simulink model "Controle_P"  (R2014a)
settings: Solver=ode45  StartTime=0.0  StopTime=1.5  RelTol=1e-3
values from neighbouring files (symbols this model uses):
  K = place(a,b,P)    [Controle_Posicao.m]
settings Model: Creator=unieerisantos  LastModifiedBy=unieerisantos
settings DataIOCC: Refine=10

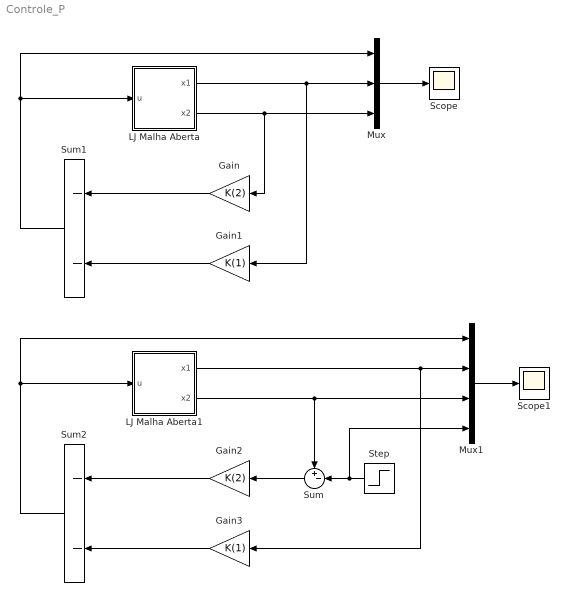
== system Controle_P ==
  Gain : Gain  Gain=K(2)
  Gain1 : Gain  Gain=K(1)
  Gain2 : Gain  Gain=K(2)
  Gain3 : Gain  Gain=K(1)
  LJ Malha Aberta : Subsystem
  LJ Malha Aberta1 : Subsystem
  Mux : Mux  Inputs=3
  Mux1 : Mux
  Scope : Scope
      settings: SaveName=ControleVcomInt
  Scope1 : Scope
  Step : Step  Time=0  After=10  SampleTime=0
  Sum : Sum  Inputs=+-|
  Sum1 : Sum  Inputs=--
  Sum2 : Sum  Inputs=--
  wires:
  LJ Malha Aberta/2("x2 ") -> Gain/1, Mux/3
  LJ Malha Aberta/1(x1) -> Gain1/1, Mux/2
  Gain/1 -> Sum1/1
  Gain1/1 -> Sum1/2
  Sum1/1 -> Mux/1, LJ Malha Aberta/1(u)
  Mux/1 -> Scope/1
  LJ Malha Aberta1/1(x1) -> Gain3/1, Mux1/2
  Gain2/1 -> Sum2/1
  Gain3/1 -> Sum2/2
  Sum2/1 -> Mux1/1, LJ Malha Aberta1/1(u)
  Mux1/1 -> Scope1/1
  LJ Malha Aberta1/2("x2 ") -> Mux1/3, Sum/1
  Sum/1 -> Gain2/1
  Step/1 -> Mux1/4, Sum/2

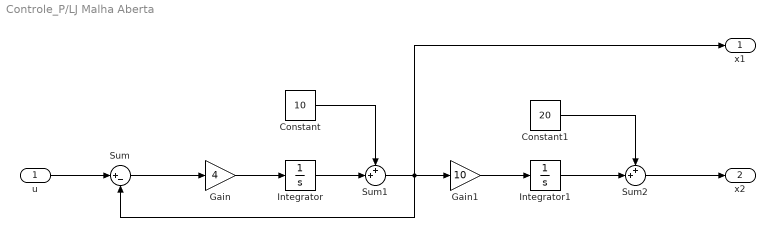
== system Controle_P/LJ Malha Aberta ==
  u : Inport
  Constant : Constant  Value=10
  Constant1 : Constant  Value=20
  Gain : Gain  Gain=4
  Gain1 : Gain  Gain=10
  Integrator : Integrator
  Integrator1 : Integrator
  Sum : Sum  Inputs=|+-
  Sum1 : Sum  Inputs=++|
  Sum2 : Sum  Inputs=++|
  x1 : Outport
  "x2 " : Outport  Port=2
  wires:
  Sum/1 -> Gain/1
  u/1 -> Sum/1
  Gain1/1 -> Integrator1/1
  Gain/1 -> Integrator/1
  Integrator/1 -> Sum1/2
  Sum1/1 -> Sum/2, x1/1, Gain1/1
  Constant/1 -> Sum1/1
  Integrator1/1 -> Sum2/2
  Constant1/1 -> Sum2/1
  Sum2/1 -> "x2 "/1

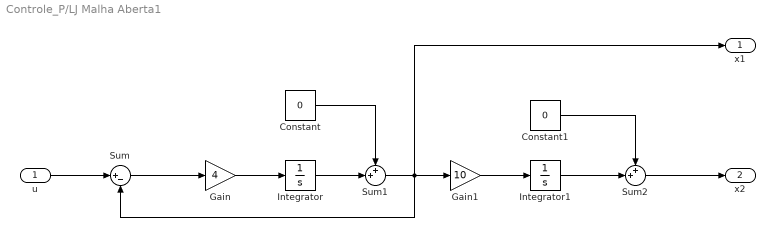
== system Controle_P/LJ Malha Aberta1 ==
  u : Inport
  Constant : Constant  Value=0
  Constant1 : Constant  Value=0
  Gain : Gain  Gain=4
  Gain1 : Gain  Gain=10
  Integrator : Integrator
  Integrator1 : Integrator
  Sum : Sum  Inputs=|+-
  Sum1 : Sum  Inputs=++|
  Sum2 : Sum  Inputs=++|
  x1 : Outport
  "x2 " : Outport  Port=2
  wires:
  Sum/1 -> Gain/1
  u/1 -> Sum/1
  Gain1/1 -> Integrator1/1
  Gain/1 -> Integrator/1
  Integrator/1 -> Sum1/2
  Sum1/1 -> Sum/2, x1/1, Gain1/1
  Constant/1 -> Sum1/1
  Integrator1/1 -> Sum2/2
  Constant1/1 -> Sum2/1
  Sum2/1 -> "x2 "/1
